simulink library "PositionDifferenceChecker"  (R2016b)
settings: Solver=VariableStepAuto  StartTime=0.0  StopTime=10.0  RelTol=1e-3
undefined symbols (not defined in the file or in its folder): maxPositionDifference
settings Model: Creator=Marc  LastModifiedBy=march

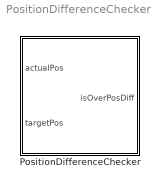
== system PositionDifferenceChecker ==
  PositionDifferenceChecker : Subsystem

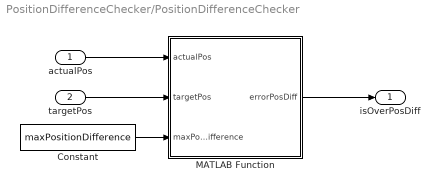
== system PositionDifferenceChecker/PositionDifferenceChecker ==
  actualPos : Inport
  targetPos : Inport  Port=2
  Constant : Constant  Value=maxPositionDifference  VectorParams1D=off  SampleTime=-1
  MATLAB Function : MATLAB Function  TreatAsAtomicUnit=on
  isOverPosDiff : Outport
  wires:
  actualPos/1 -> MATLAB Function/1(actualPos)
  MATLAB Function/1(errorPosDiff) -> isOverPosDiff/1
  targetPos/1 -> MATLAB Function/2(targetPos)
  Constant/1 -> MATLAB Function/3(maxPositionDifference)

== matlab function PositionDifferenceChecker/MATLAB Function ==
  data: actualPos input; targetPos input; errorPosDiff output; maxPositionDifference input
function errorPosDiff = fcn(actualPos, targetPos, maxPositionDifference)
persistent samplesTooSlow;
if(isempty(samplesTooSlow))
    samplesTooSlow = 0;
end
if any(abs(targetPos - actualPos) > maxPositionDifference) % any so vector input still triggers error
    samplesTooSlow = samplesTooSlow + 1;
else
    samplesTooSlow = 0;
end

errorPosDiff = samplesTooSlow > 5; % as too filter out weird actual positions and state transition problems
end
